simulink model "phase1_baseline_sampling_jitter"  (R2026a)
settings: Solver=FixedStepAuto
model workspace (MAT data in the model file):
  tau = 0
undefined symbols (not defined in the file): simulationParams
settings Model: Creator=rayyu  LastModifiedBy=rayyu

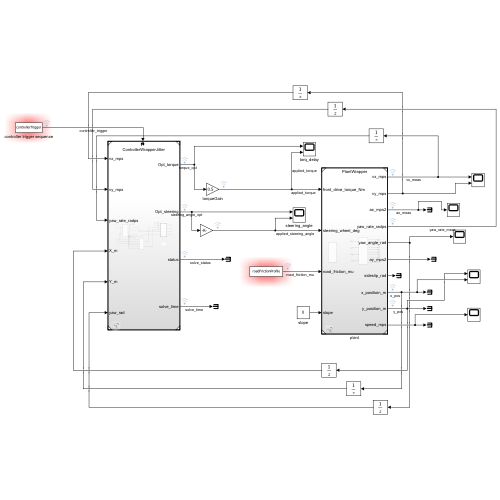
[thumbnail: Simulink's stored preview of the top-level diagram]
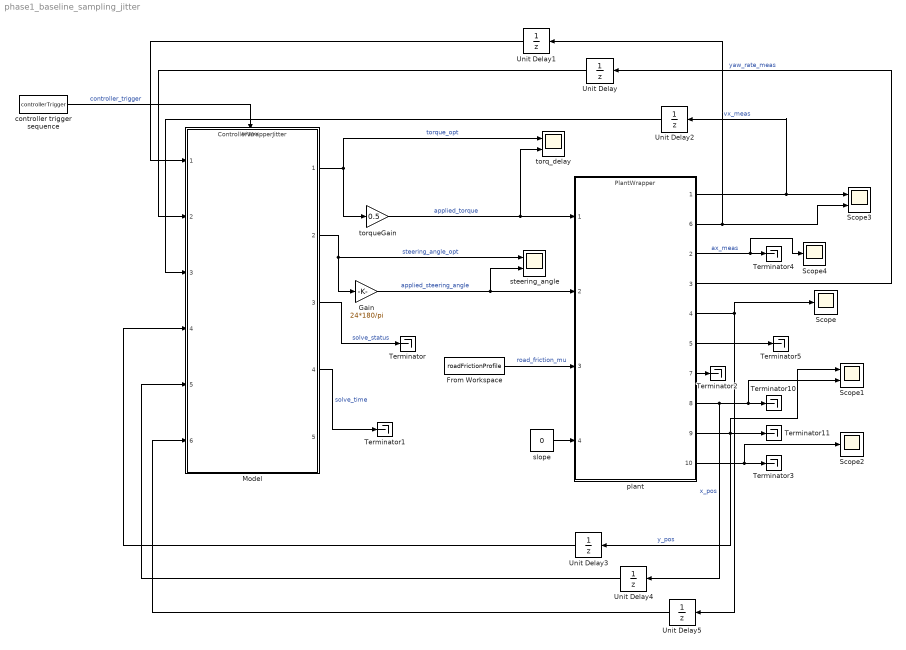
== system phase1_baseline_sampling_jitter ==
  From Workspace : FromWorkspace  VariableName=roadFrictionProfile  SampleTime=simulationParams.Ts_s  Interpolate=off  OutputAfterFinalValue=Holding final value
  Gain : Gain  Gain=24*180/pi
  Model : ModelReference  ModelNameDialog=ControllerWrapperJitter.slx  SimulationMode=Normal  ModelReferenceVersion=1.44  TriggerPortName=Trigger  TriggerPortTriggerType=rising
  Scope : Scope
      settings: ActiveDisplayYMinimum=-1  ActiveDisplayYMaximum=1  DataLoggingVariableName=ScopeData4
  Scope1 : Scope  NumInputPorts=2
      settings: ActiveDisplayYMinimum=-21.988383930357102  ActiveDisplayYMaximum=153.74859051736982
  Scope2 : Scope
      settings: ActiveDisplayYMinimum=0  ActiveDisplayYMaximum=2.8635963178323579E-22  DataLoggingVariableName=ScopeData2
  Scope3 : Scope  NumInputPorts=2
      settings: ActiveDisplayYMinimum=-10.190231160058753  ActiveDisplayYMaximum=56.68780346222875  DataLoggingVariableName=ScopeData5
  Scope4 : Scope
      settings: ActiveDisplayYMinimum=-268098.75332313258  ActiveDisplayYMaximum=381760.8424542984  DataLoggingVariableName=ScopeData6
  Terminator{,1..5,10..11} (8 alike) : Terminator
  Unit Delay{,1..5} (6 alike) : UnitDelay  SampleTime=-1
  controller trigger sequence : FromWorkspace  VariableName=controllerTrigger  SampleTime=-1  Interpolate=off  OutputAfterFinalValue=Holding final value
  plant : ModelReference  ModelNameDialog=PlantWrapper.slx  SimulationMode=Normal  ModelReferenceVersion=1.22
      settings: PortSchema="{\"entries\":[{\"content\":{\"sides\":[{\"content\":{\"connectorIds\":[\"In1\",\"In2\",\"In3\",\"In4\"]},\"type\":\"ConnectorPlacement.EquallySpacedRectSide\",\"uuid\":\"bf665537-3fd8-4fa0-88a8-2cb308153754\"},{\"content\":{\"connectorIds\":[\"Out1\",\"Out6\",\"Out2\",\"Out3\",\"Out4\",\"Out5\",\"Out7\",\"Out8\",\"Out9\",\"Out10\"],\"side\":\"RIGHT\"},\"type\":\"ConnectorPlacement.EquallySpacedRectSide\",\"uuid\":\"a274990e-adc2-49b8-8679-a2f39e53ce6e\"},{\"content\":{\"side\":\"TOP\"},\"type\":\"ConnectorPlacement.EquallySpacedRectSide\",\"uuid\":\"963f9bff-e020-46b1-9958-cad0758083aa\"}]},\"type\":\"ConnectorPlacement.EquallySpacedConnector\",\"uuid\":\"fb8d0fca-1617-49ee-84dd-83e8b757a297\"}],\"packageUris\":[\"http://schema.mathworks.com/mf0/Connector/R2020b\"],\"version\":\"1.0\"}"
  slope : Constant  Value=0
  steering_angle : Scope  NumInputPorts=2
      settings: ActiveDisplayYMinimum=-183.84826338257844  ActiveDisplayYMaximum=186.50850743591388  DataLoggingVariableName=ScopeData3
  torq_delay : Scope  NumInputPorts=2
      settings: ActiveDisplayYMinimum=119.57395931342806  ActiveDisplayYMaximum=269.14536264631744  DataLoggingVariableName=ScopeData7
  torqueGain : Gain  Gain=0.5
  wires:
  plant/4 -> Unit Delay5/1, Scope/1
  plant/6 -> Unit Delay1/1, Scope3/2
  plant/1 -> Scope3/1, Unit Delay2/1  "vx_meas"
  plant/7 -> Terminator2/1
  slope/1 -> plant/4
  plant/3 -> Unit Delay/1  "yaw_rate_meas"
  plant/2 -> Scope4/1, Terminator4/1  "ax_meas"
  plant/10 -> Scope2/1, Terminator3/1
  From Workspace/1 -> plant/3  "road_friction_mu"
  plant/8 -> Unit Delay4/1, Scope1/2, Terminator10/1  "x_pos"
  plant/5 -> Terminator5/1
  plant/9 -> Unit Delay3/1, Scope1/1, Terminator11/1  "y_pos"
  torqueGain/1 -> torq_delay/2, plant/1  "applied_torque"
  Gain/1 -> steering_angle/2, plant/2  "applied_steering_angle"
  Model/2 -> steering_angle/1, Gain/1  "steering_angle_opt"
  Model/1 -> torqueGain/1, torq_delay/1  "torque_opt"
  Unit Delay1/1 -> Model/1
  Unit Delay/1 -> Model/2
  Unit Delay2/1 -> Model/3
  Unit Delay3/1 -> Model/4
  Unit Delay4/1 -> Model/5
  Unit Delay5/1 -> Model/6
  Model/3 -> Terminator/1  "solve_status"
  Model/4 -> Terminator1/1  "solve_time"
  controller trigger sequence/1 -> Model/Trigger  "controller_trigger"
